simulink model "CompassPID"  (R2014b)
settings: Solver=FixedStepDiscrete  StartTime=0.0  StopTime=10.0  RelTol=1e-3
libraries: arduinolib x2, SkywardBLIMP x1, simulink x1
settings Model: ExtModeTrigDuration=2  Creator=Francescodario  LastModifiedBy=Francescodario
settings OptimizationCC: OptimizeModelRefInitCode=on  LifeSpan=1
settings DebuggingCC: UnderspecifiedInitializationDetection=Classic  MergeDetectMultiDrivingBlocksExec=none  SolverPrmCheckMsg=none
settings HardwareCC: ProdBitPerInt=16  ProdBitPerPointer=8  ProdIntDivRoundTo=Zero  ProdEndianess=LittleEndian  ProdWordSize=8  ProdHWDeviceType=Atmel->AVR
settings RTWCC: SystemTargetFile=realtime.tlc  GenerateMakefile=off  TemplateMakefile=realtime.tmf  Description=Run on Target Hardware  RTWVerbose=off  ProcessScript=realtime_make_rtw_hook
settings STFCustomTargetCC: TargetLibSuffix=.a  GenerateSampleERTMain=on  ERTCustomFileBanners=on  SupportNonInlinedSFcns=off  SupportVariableSizeSignals=on  MATLABClassNameForMDSCustomization=Simulink.SoftwareTarget.ERTCustomization  GRTInterface=off  SystemTargetFile=realtime.tlc
settings ERTTargetCC: GenerateSampleERTMain=on  ParMdlRefBuildCompliant=off  CompOptLevelCompliant=off  ConcurrentExecutionCompliant=off  CombineOutputUpdateFcns=off  ERTFirstTimeCompliant=off  SupportContinuousTime=on  SupportVariableSizeSignals=on  ModelStepFunctionPrototypeControlCompliant=off  CPPClassGenCompliant=off  ExtModeTransport=3  ExtModeMexFile=ext_serial_win32_comm  ExtModeMexArgs=0 1 9600  InlinedParameterPlacement=NonHierarchical  ERTSrcFileBannerTemplate=realtime_code_template.cgt  ERTHdrFileBannerTemplate=realtime_code_template.cgt  ERTDataSrcFileTemplate=realtime_code_template.cgt  ERTDataHdrFileTemplate=realtime_code_template.cgt  ERTCustomFileTemplate=realtime_file_process.tlc

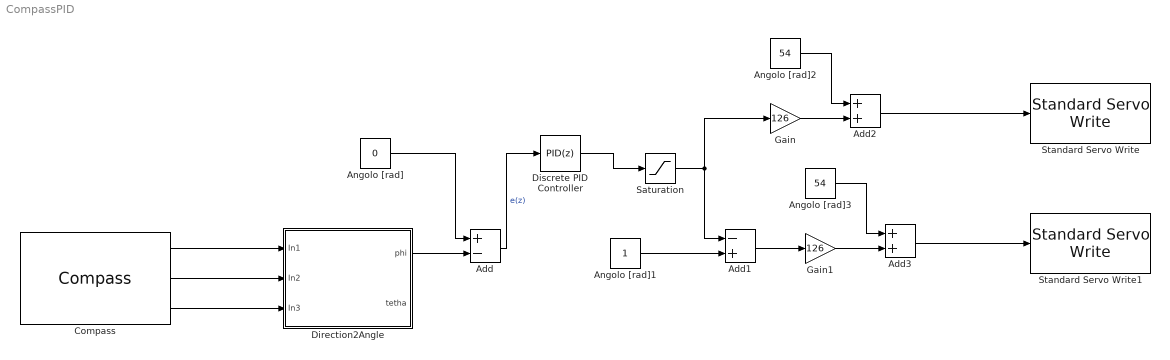
== system CompassPID ==
  Add : Sum  Inputs=+-
  Add1 : Sum  Inputs=-+
  Add2 : Sum
  Add3 : Sum
  Angolo [rad] : Constant  Value=0  SampleTime=0.1
  Angolo [rad]1 : Constant  SampleTime=0.1
  Angolo [rad]2 : Constant  Value=54  SampleTime=0.1
  Angolo [rad]3 : Constant  Value=54  SampleTime=0.1
  Compass : SkywardBLIMP/Compass
  Direction2Angle : Subsystem
  Discrete PID Controller : simulink/Continuous/PID Controller  Controller=PID  TimeDomain=Discrete-time  SampleTime=-1  IntegratorMethod=Trapezoidal  FilterMethod=Forward Euler  Form=Parallel  P=1.5  I=0.2  D=2  N=100  InitialConditionSource=internal  InitialConditionForIntegrator=0  InitialConditionForFilter=0  ExternalReset=none  LimitOutput=off  UpperSaturationLimit=inf  LowerSaturationLimit=-inf  LinearizeAsGain=off  AntiWindupMode=none  Kb=1  TrackingMode=off  Kt=1  PParamMin=[]  PParamMax=[]  IParamMin=[]  IParamMax=[]  DParamMin=[]  DParamMax=[]  NParamMin=[]  NParamMax=[]  KbParamMin=[]  KbParamMax=[]  KtParamMin=[]  KtParamMax=[]  POutMin=[]  POutMax=[]  IOutMin=[]  IOutMax=[]  DOutMin=[]  DOutMax=[]  NOutMin=[]  NOutMax=[]  KbOutMin=[]  KbOutMax=[]  KtOutMin=[]  KtOutMax=[]  IntegratorOutMin=[]  IntegratorOutMax=[]  FilterOutMin=[]  FilterOutMax=[]  SumOutMin=[]  SumOutMax=[]  SumI1OutMin=[]  SumI1OutMax=[]  SumI2OutMin=[]  SumI2OutMax=[]  SumI3OutMin=[]  SumI3OutMax=[]  SumDOutMin=[]  SumDOutMax=[]  SaturationOutMin=[]  SaturationOutMax=[]  IntegratorContinuousStateAttributes=''  IntegratorStateMustResolveToSignalObject=off  IntegratorRTWStateStorageClass=Auto  FilterContinuousStateAttributes=''  FilterStateMustResolveToSignalObject=off  FilterRTWStateStorageClass=Auto  DifferentiatorICPrevScaledInput=0  DifferentiatorOutMin=[]  DifferentiatorOutMax=[]  UseFilter=on
  Gain : Gain  Gain=126
  Gain1 : Gain  Gain=126
  Saturation : Saturate  UpperLimit=1  LowerLimit=0
  Standard Servo Write : arduinolib/Standard Servo Write  pinNumber=4  blockPlatform=arduino
  Standard Servo Write1 : arduinolib/Standard Servo Write  pinNumber=9  blockPlatform=arduino
  wires:
  Compass/1 -> Direction2Angle/1(In1)
  Compass/2 -> Direction2Angle/2(In2)
  Compass/3 -> Direction2Angle/3(In3)
  Saturation/1 -> Add1/1, Gain/1
  Add1/1 -> Gain1/1
  Direction2Angle/1(phi) -> Add/2
  Angolo [rad]/1 -> Add/1
  Angolo [rad]1/1 -> Add1/2
  Add/1 -> Discrete PID Controller/1  "e(z)"
  Discrete PID Controller/1 -> Saturation/1
  Gain/1 -> Add2/2
  Angolo [rad]2/1 -> Add2/1
  Gain1/1 -> Add3/2
  Angolo [rad]3/1 -> Add3/1
  Add2/1 -> Standard Servo Write/1
  Add3/1 -> Standard Servo Write1/1

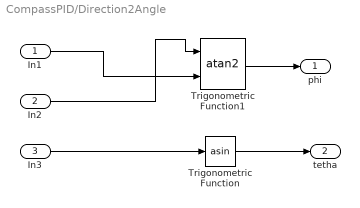
== system CompassPID/Direction2Angle ==
  In1 : Inport
  In2 : Inport  Port=2
  In3 : Inport  Port=3
  Trigonometric Function : Trigonometry  Operator=asin
  Trigonometric Function1 : Trigonometry  Operator=atan2
  phi : Outport
  tetha : Outport  Port=2
  wires:
  In1/1 -> Trigonometric Function1/2
  Trigonometric Function1/1 -> phi/1
  In3/1 -> Trigonometric Function/1
  In2/1 -> Trigonometric Function1/1
  Trigonometric Function/1 -> tetha/1
